simulink library "powerwindowlibsa"  (Simulink 6.0)
settings: Solver=ode45  SolverMode=SingleTasking  StartTime=0.0  StopTime=10.0  RelTol=1e-3
InitFcn:
  | powericon('psbinitsys',bdroot);
libraries: fixpt_lib_4 x2, simulink x2, powerwindowlibsa x1
settings Model: Creator=The MathWorks Inc.  LastModifiedBy=batserve  ExtModeAutoUpdateStatusClock=off
settings OptimizationCC: BooleanDataType=off
settings DebuggingCC: CheckExecutionContextPreStartOutputMsg=on  CheckExecutionContextRuntimeOutputMsg=on  SolverPrmCheckMsg=none
settings HardwareCC: TargetUnknown=on

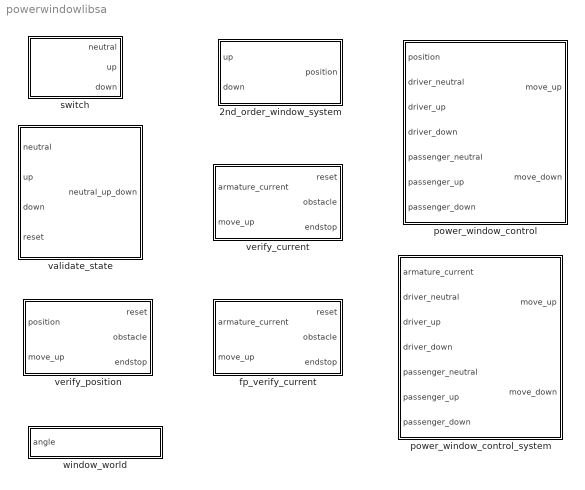
== system powerwindowlibsa ==
  2nd_order_window_system : Subsystem  PropExecContextAcrossSSBoundary=on
  fp_verify_current : Subsystem  AncestorBlock=powerwindowlibsa/verify_current  PropExecContextAcrossSSBoundary=on
  power_window_control : Subsystem  PropExecContextAcrossSSBoundary=on
  power_window_control_system : Subsystem  PropExecContextAcrossSSBoundary=on
  switch : Subsystem  PropExecContextAcrossSSBoundary=on
  validate_state : Subsystem  PropExecContextAcrossSSBoundary=on
  verify_current : Subsystem  AncestorBlock=powerwindowlibsa/power_window_control_system/detect_obstacle_endstop  PropExecContextAcrossSSBoundary=on
  verify_position : Subsystem  AncestorBlock=powerwindowlibsa/detect_obstacle_endstop  PropExecContextAcrossSSBoundary=on
  window_world : Subsystem  AncestorBlock=powerwindowlibsa/window_world  PropExecContextAcrossSSBoundary=on
      settings: OpenFcn=open_system([gcs '/window_world/VR Sink']);
      mask Display: disp(sprintf('Double-click to view scene'))

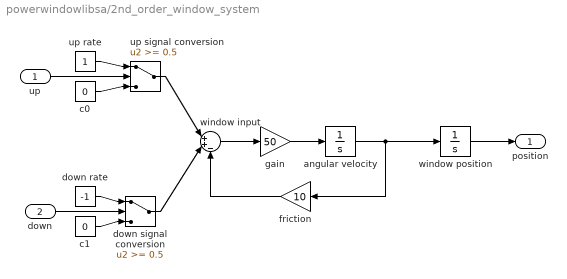
== system powerwindowlibsa/2nd_order_window_system ==
  up : Inport  Port=1  LatchInput=off
  down : Inport  Port=2  LatchInput=off
  angular velocity : Integrator
  c0 : Constant  Value=0
  c1 : Constant  Value=0
  down rate : Constant  Value=-1
  down signal conversion : Switch  Threshold=0.5  SaturateOnIntegerOverflow=on  InputSameDT=on
  friction : Gain  Orientation=left  Gain=10  SaturateOnIntegerOverflow=on
  gain : Gain  Gain=50  SaturateOnIntegerOverflow=on
  up rate : Constant
  up signal conversion : Switch  Threshold=0.5  SaturateOnIntegerOverflow=on  InputSameDT=on
  window input : Sum  Inputs=|++-  SaturateOnIntegerOverflow=on  InputSameDT=on
  window position : Integrator
  position : Outport
  wires:
  down/1 -> down signal conversion/2
  window position/1 -> position/1
  up/1 -> up signal conversion/2
  up rate/1 -> up signal conversion/1
  c0/1 -> up signal conversion/3
  down rate/1 -> down signal conversion/1
  c1/1 -> down signal conversion/3
  up signal conversion/1 -> window input/1
  down signal conversion/1 -> window input/2
  window input/1 -> gain/1
  gain/1 -> angular velocity/1
  angular velocity/1 -> friction/1, window position/1
  friction/1 -> window input/3

== system powerwindowlibsa/fp_verify_current ==
  armature_current : Inport  Port=1  LatchInput=off
  move_up : Inport  Port=2  LatchInput=off
  detect_endstop : Subsystem  PropExecContextAcrossSSBoundary=on
  detect_obstacle : Subsystem  PropExecContextAcrossSSBoundary=on
  either : Logic  Operator=OR
  process_current : Subsystem  PropExecContextAcrossSSBoundary=on
  reset : Outport
  obstacle : Outport  Port=2
  endstop : Outport  Port=3
  wires:
  armature_current/1 -> process_current/1(raw_current)
  detect_obstacle/1(obstacle) -> either/1, obstacle/1
  detect_endstop/1(endstop) -> endstop/1, either/2
  either/1 -> reset/1
  move_up/1 -> detect_obstacle/1(move_up)
  process_current/1(processed_current) -> detect_obstacle/2(armature_current), detect_endstop/1(armature_current)

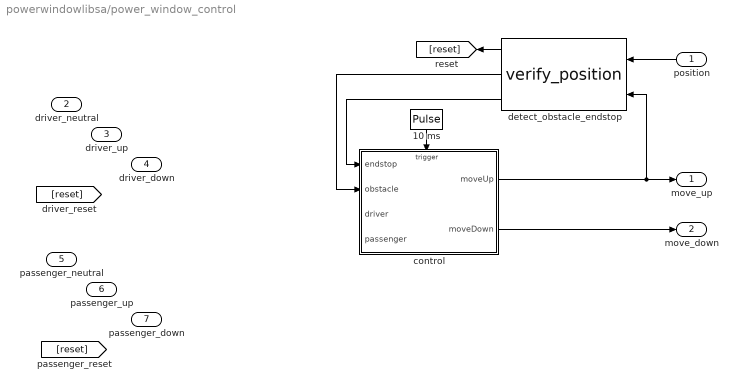
== system powerwindowlibsa/power_window_control ==
  position : Inport  Orientation=left  Port=1  LatchInput=off
  driver_neutral : Inport  Port=2  LatchInput=off
  driver_up : Inport  Port=3  LatchInput=off
  driver_down : Inport  Port=4  LatchInput=off
  passenger_neutral : Inport  Port=5  LatchInput=off
  passenger_up : Inport  Port=6  LatchInput=off
  passenger_down : Inport  Port=7  LatchInput=off
  10 ms : DiscretePulseGenerator  Orientation=down  SampleTime=10e-3
  control : Stateflow chart  TreatAsAtomicUnit=on  PropExecContextAcrossSSBoundary=on
  detect_obstacle_endstop : powerwindowlibsa/verify_position  Orientation=left  AncestorBlock=powerwindowlibsa/detect_obstacle_endstop  SimViewingDevice=off  DataTypeOverride=UseLocalSettings  MinMaxOverflowLogging=UseLocalSettings
      settings: Permissions=ReadWrite  RTWFcnNameOpts=Auto  RTWFileNameOpts=Auto
  move_up : Outport
  move_down : Outport  Port=2
  wires:
  control/2(moveDown) -> move_down/1
  control/1(moveUp) -> move_up/1, detect_obstacle_endstop/2
  10 ms/1 -> control/Trigger
  position/1 -> detect_obstacle_endstop/1
  detect_obstacle_endstop/1 -> [reset]
  detect_obstacle_endstop/3 -> control/1(endstop)
  detect_obstacle_endstop/2 -> control/2(obstacle)

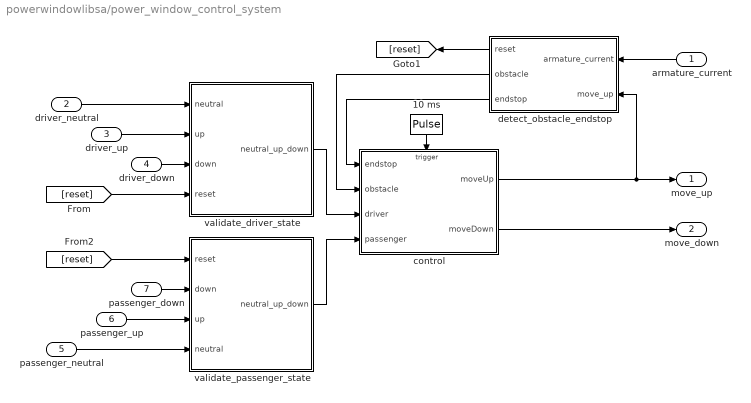
== system powerwindowlibsa/power_window_control_system ==
  armature_current : Inport  Orientation=left  Port=1  LatchInput=off
  driver_neutral : Inport  Port=2  LatchInput=off
  driver_up : Inport  Port=3  LatchInput=off
  driver_down : Inport  Port=4  LatchInput=off
  passenger_neutral : Inport  Port=5  LatchInput=off
  passenger_up : Inport  Port=6  LatchInput=off
  passenger_down : Inport  Port=7  LatchInput=off
  10 ms : DiscretePulseGenerator  Orientation=down  PulseType=Time based  Period=1e-2  SampleTime=1e-3
  control : Stateflow chart  TreatAsAtomicUnit=on  PropExecContextAcrossSSBoundary=on
  detect_obstacle_endstop : Subsystem  Orientation=left  PropExecContextAcrossSSBoundary=on
  validate_driver_state : Subsystem  PropExecContextAcrossSSBoundary=on
  validate_passenger_state : Subsystem  PropExecContextAcrossSSBoundary=on
  move_up : Outport
  move_down : Outport  Port=2
  wires:
  armature_current/1 -> detect_obstacle_endstop/1(armature_current)
  control/2(moveDown) -> move_down/1
  control/1(moveUp) -> detect_obstacle_endstop/2(move_up), move_up/1
  detect_obstacle_endstop/3(endstop) -> control/1(endstop)
  detect_obstacle_endstop/2(obstacle) -> control/2(obstacle)
  validate_passenger_state/1(neutral_up_down) -> control/4(passenger)
  validate_driver_state/1(neutral_up_down) -> control/3(driver)
  10 ms/1 -> control/Trigger
  detect_obstacle_endstop/1(reset) -> [reset]
  [reset] -> validate_passenger_state/1(reset)
  passenger_down/1 -> validate_passenger_state/2(down)
  passenger_up/1 -> validate_passenger_state/3(up)
  passenger_neutral/1 -> validate_passenger_state/4(neutral)
  driver_down/1 -> validate_driver_state/3(down)
  driver_up/1 -> validate_driver_state/2(up)
  driver_neutral/1 -> validate_driver_state/1(neutral)
  [reset] -> validate_driver_state/4(reset)

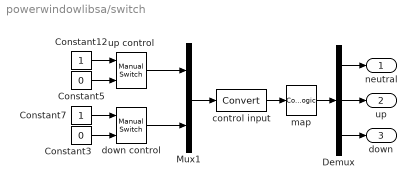
== system powerwindowlibsa/switch ==
  Constant12 : Constant
  Constant3 : Constant  Value=0
  Constant5 : Constant  Value=0
  Constant7 : Constant
  Demux : Demux  Outputs=3
  Mux1 : Mux  Inputs=2
  control input : DataTypeConversion  OutDataTypeMode=boolean  SaturateOnIntegerOverflow=on  RndMeth=Zero
  down control : simulink/Signal Routing/Manual Switch  sw=0  action=0
  map : CombinatorialLogic  TruthTable=[1 0 0;0 0 1;0 1 0;1 0 0]
  up control : simulink/Signal Routing/Manual Switch  sw=0  action=0
  neutral : Outport
  up : Outport  Port=2
  down : Outport  Port=3
  wires:
  Demux/3 -> down/1
  Demux/2 -> up/1
  Demux/1 -> neutral/1
  map/1 -> Demux/1
  up control/1 -> Mux1/1
  Mux1/1 -> control input/1
  down control/1 -> Mux1/2
  Constant3/1 -> down control/2
  Constant7/1 -> down control/1
  Constant5/1 -> up control/2
  Constant12/1 -> up control/1
  control input/1 -> map/1

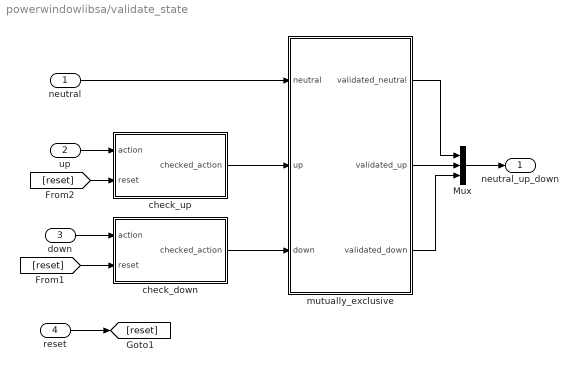
== system powerwindowlibsa/validate_state ==
  neutral : Inport  Port=1  LatchInput=off
  up : Inport  Port=2  LatchInput=off
  down : Inport  Port=3  LatchInput=off
  reset : Inport  Port=4  LatchInput=off
  Mux : Mux  Inputs=3
  check_down : Subsystem  PropExecContextAcrossSSBoundary=on
  check_up : Subsystem  PropExecContextAcrossSSBoundary=on
  mutually_exclusive : Subsystem  PropExecContextAcrossSSBoundary=on
  neutral_up_down : Outport
  wires:
  check_down/1(checked_action) -> mutually_exclusive/3(down)
  mutually_exclusive/3(validated_down) -> Mux/3
  mutually_exclusive/2(validated_up) -> Mux/2
  mutually_exclusive/1(validated_neutral) -> Mux/1
  down/1 -> check_down/1(action)
  up/1 -> check_up/1(action)
  neutral/1 -> mutually_exclusive/1(neutral)
  check_up/1(checked_action) -> mutually_exclusive/2(up)
  [reset] -> check_up/2(reset)
  [reset] -> check_down/2(reset)
  reset/1 -> [reset]
  Mux/1 -> neutral_up_down/1

== system powerwindowlibsa/verify_current ==
  armature_current : Inport  Port=1  LatchInput=off
  move_up : Inport  Port=2  LatchInput=off
  detect_endstop : Subsystem  PropExecContextAcrossSSBoundary=on
  detect_obstacle : Subsystem  PropExecContextAcrossSSBoundary=on
  either : Logic  Operator=OR
  process_current : Subsystem  PropExecContextAcrossSSBoundary=on
  reset : Outport
  obstacle : Outport  Port=2
  endstop : Outport  Port=3
  wires:
  process_current/1(processed_current) -> detect_endstop/1(armature_current), detect_obstacle/2(armature_current)
  move_up/1 -> detect_obstacle/1(move_up)
  either/1 -> reset/1
  detect_endstop/1(endstop) -> either/2, endstop/1
  detect_obstacle/1(obstacle) -> obstacle/1, either/1
  armature_current/1 -> process_current/1(raw_current)

== system powerwindowlibsa/verify_position ==
  position : Inport  Port=1  LatchInput=off
  move_up : Inport  Port=2  LatchInput=off
  detect_endstop : Subsystem  PropExecContextAcrossSSBoundary=on
  detect_obstacle : Subsystem  PropExecContextAcrossSSBoundary=on
  either : Logic  Operator=OR
  reset : Outport
  obstacle : Outport  Port=2
  endstop : Outport  Port=3
  wires:
  move_up/1 -> detect_obstacle/1(move_up)
  position/1 -> detect_endstop/1(position), detect_obstacle/2(position)
  either/1 -> reset/1
  detect_endstop/1(endstop) -> either/2, endstop/1
  detect_obstacle/1(obstacle) -> obstacle/1, either/1

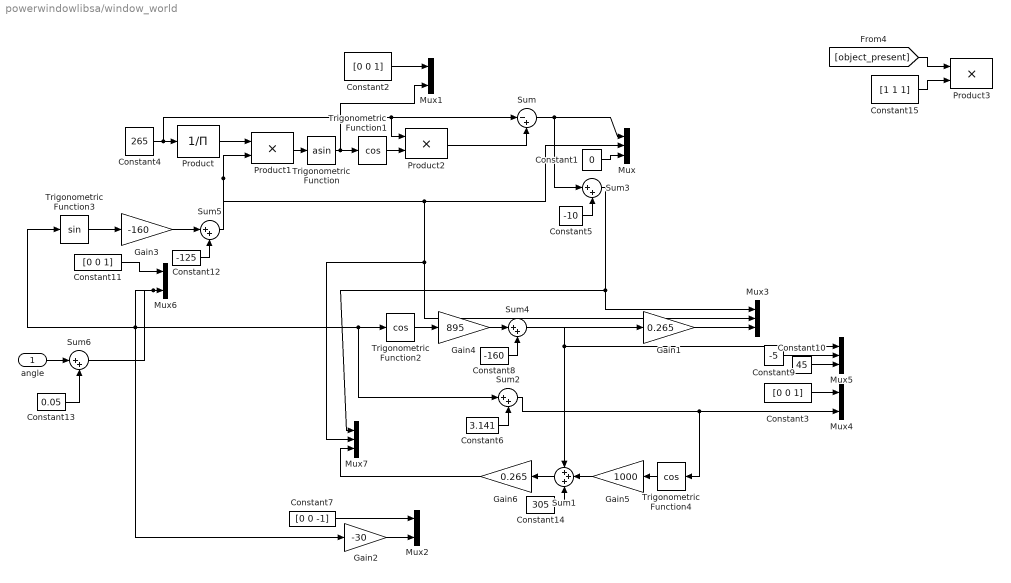
== system powerwindowlibsa/window_world ==
  angle : Inport  Port=1  LatchInput=off
  Constant1 : Constant  Value=0
  Constant10 : Constant  Value=45
  Constant11 : Constant  Value=[0 0 1]
  Constant12 : Constant  Value=-125
  Constant13 : Constant  Value=0.05
  Constant14 : Constant  Value=305
  Constant15 : Constant  Value=[1 1 1]
  Constant2 : Constant  Value=[0 0 1]
  Constant3 : Constant  Value=[0 0 1]
  Constant4 : Constant  Value=265
  Constant5 : Constant  Value=-10
  Constant6 : Constant  Value=3.141
  Constant7 : Constant  Value=[0 0 -1]
  Constant8 : Constant  Value=-160
  Constant9 : Constant  Value=-5
  Gain1 : Gain  Gain=0.265  SaturateOnIntegerOverflow=on
  Gain2 : Gain  Gain=-30  SaturateOnIntegerOverflow=on
  Gain3 : Gain  Gain=-160  SaturateOnIntegerOverflow=on
  Gain4 : Gain  Gain=895  SaturateOnIntegerOverflow=on
  Gain5 : Gain  Orientation=left  Gain=1000  SaturateOnIntegerOverflow=on
  Gain6 : Gain  Orientation=left  Gain=0.265  SaturateOnIntegerOverflow=on
  Mux{,3,5,7} (4 alike) : Mux  Inputs=3
  Mux{1..2,4,6} (4 alike) : Mux  Inputs=2
  Product : Product  Inputs=/  SaturateOnIntegerOverflow=on  InputSameDT=on
  Product1 : Product  SaturateOnIntegerOverflow=on  InputSameDT=on
  Product2 : Product  SaturateOnIntegerOverflow=on  InputSameDT=on
  Product3 : Product  SaturateOnIntegerOverflow=on  InputSameDT=on
  Sum : Sum  Inputs=|-+  SaturateOnIntegerOverflow=on  InputSameDT=on
  Sum1 : Sum  Orientation=left  Inputs=+++  SaturateOnIntegerOverflow=on  InputSameDT=on
  Sum{2..6} (5 alike) : Sum  Inputs=|++  SaturateOnIntegerOverflow=on  InputSameDT=on
  Trigonometric Function : Trigonometry  Operator=asin
  Trigonometric Function1 : Trigonometry  Operator=cos
  Trigonometric Function2 : Trigonometry  Operator=cos
  Trigonometric Function3 : Trigonometry
  Trigonometric Function4 : Trigonometry  Orientation=left  Operator=cos
  wires:
  Constant5/1 -> Sum3/2
  Sum3/1 -> Mux7/1, Mux3/1
  Constant14/1 -> Sum1/3
  Gain6/1 -> Mux7/3
  Sum1/1 -> Gain6/1
  Gain5/1 -> Sum1/2
  Trigonometric Function4/1 -> Gain5/1
  Gain1/1 -> Mux3/3
  Constant7/1 -> Mux2/1
  Gain2/1 -> Mux2/2
  Sum5/1 -> Mux7/2, Mux3/2, Mux/2, Product1/2
  Gain3/1 -> Sum5/1
  Constant12/1 -> Sum5/2
  Constant11/1 -> Mux6/1
  Trigonometric Function3/1 -> Gain3/1
  Constant8/1 -> Sum4/2
  Sum4/1 -> Sum1/1, Mux5/1, Gain1/1
  Gain4/1 -> Sum4/1
  Trigonometric Function2/1 -> Gain4/1
  Constant10/1 -> Mux5/3
  Constant9/1 -> Mux5/2
  Constant6/1 -> Sum2/2
  Sum2/1 -> Trigonometric Function4/1, Mux4/2
  Constant3/1 -> Mux4/1
  Sum/1 -> Sum3/1, Mux/1
  Product2/1 -> Sum/2
  Trigonometric Function1/1 -> Product2/2
  Trigonometric Function/1 -> Mux1/2, Trigonometric Function1/1
  Product1/1 -> Trigonometric Function/1
  Product/1 -> Product1/1
  Constant4/1 -> Sum/1, Product2/1, Product/1
  Constant2/1 -> Mux1/1
  Constant1/1 -> Mux/3
  Sum6/1 -> Mux6/2, Gain2/1, Trigonometric Function2/1, Sum2/1, Trigonometric Function3/1
  angle/1 -> Sum6/1
  Constant13/1 -> Sum6/2
  Constant15/1 -> Product3/2
  [object_present] -> Product3/1

== system powerwindowlibsa/fp_verify_current/detect_endstop ==
  armature_current : Inport  Port=1  LatchInput=off
  current_limit : fixpt_lib_4/Logic & Comparison/Compare To Constant  relop=>  const=15
  passenger control : DataTypeConversion  OutDataTypeMode=boolean  SaturateOnIntegerOverflow=on  RndMeth=Zero
  endstop : Outport
  wires:
  passenger control/1 -> endstop/1
  current_limit/1 -> passenger control/1
  armature_current/1 -> current_limit/1

== system powerwindowlibsa/fp_verify_current/detect_obstacle ==
  move_up : Inport  Orientation=left  Port=1  LatchInput=off
  armature_current : Inport  Port=2  LatchInput=off
  10 ms : DiscretePulseGenerator  Orientation=down  SampleTime=10e-3
  Multiply : Product  Orientation=up  Inputs=**  OutDataType=sfix(8)  OutScaling=2^-5
  break dependency : UnitDelay  Orientation=left  SampleTime=0.01
  current_limit : fixpt_lib_4/Logic & Comparison/Compare To Constant  relop=>  const=1.1
  delay_detection : Stateflow chart  Orientation=left  TreatAsAtomicUnit=on  PropExecContextAcrossSSBoundary=on
  passenger control : DataTypeConversion  Orientation=up  OutDataTypeMode=boolean  SaturateOnIntegerOverflow=on  RndMeth=Zero
  obstacle : Outport  Orientation=up
  wires:
  passenger control/1 -> obstacle/1
  break dependency/1 -> delay_detection/1(move_up)
  10 ms/1 -> delay_detection/Trigger
  Multiply/1 -> passenger control/1
  move_up/1 -> break dependency/1
  armature_current/1 -> current_limit/1
  delay_detection/1(detect) -> Multiply/2
  current_limit/1 -> Multiply/1

== system powerwindowlibsa/fp_verify_current/process_current ==
  raw_current : Inport  Port=1  LatchInput=off
  3.5 / (2^(bits-1)) : Gain  Gain=0.02734375  ParameterDataType=sfix( 8 )  ParameterScaling=2^-12  OutDataTypeMode=Specify via dialog  OutScaling=2^-6
  Abs : Abs
  gain : Gain  Gain=5  ParameterDataType=sfix( 8 )  ParameterScaling=2^-4  OutDataTypeMode=Specify via dialog  OutScaling=2^-5
  processed_current : Outport
  wires:
  raw_current/1 -> 3.5 / (2^(bits-1))/1
  Abs/1 -> processed_current/1
  gain/1 -> Abs/1
  3.5 / (2^(bits-1))/1 -> gain/1

== system powerwindowlibsa/power_window_control_system/detect_obstacle_endstop ==
  armature_current : Inport  Port=1  LatchInput=off
  move_up : Inport  Port=2  LatchInput=off
  Abs : Abs  SaturateOnIntegerOverflow=on
  detect_endstop : Subsystem  PropExecContextAcrossSSBoundary=on
  detect_obstacle : Subsystem  PropExecContextAcrossSSBoundary=on
  either : Logic  Operator=OR
  reset : Outport
  obstacle : Outport  Port=2
  endstop : Outport  Port=3
  wires:
  detect_obstacle/1(obstacle) -> either/1, obstacle/1
  detect_endstop/1(endstop) -> endstop/1, either/2
  either/1 -> reset/1
  armature_current/1 -> Abs/1
  move_up/1 -> detect_obstacle/1(move_up)
  Abs/1 -> detect_obstacle/2(armature_current), detect_endstop/1(armature_current)

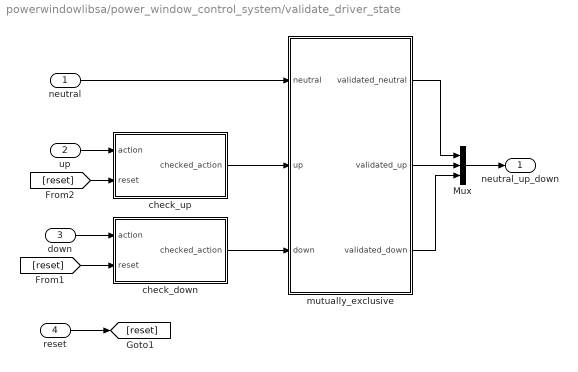
== system powerwindowlibsa/power_window_control_system/validate_driver_state ==
  neutral : Inport  Port=1  LatchInput=off
  up : Inport  Port=2  LatchInput=off
  down : Inport  Port=3  LatchInput=off
  reset : Inport  Port=4  LatchInput=off
  Mux : Mux  Inputs=3
  check_down : Subsystem  PropExecContextAcrossSSBoundary=on
  check_up : Subsystem  PropExecContextAcrossSSBoundary=on
  mutually_exclusive : Subsystem  PropExecContextAcrossSSBoundary=on
  neutral_up_down : Outport
  wires:
  check_down/1(checked_action) -> mutually_exclusive/3(down)
  mutually_exclusive/3(validated_down) -> Mux/3
  mutually_exclusive/2(validated_up) -> Mux/2
  mutually_exclusive/1(validated_neutral) -> Mux/1
  down/1 -> check_down/1(action)
  up/1 -> check_up/1(action)
  neutral/1 -> mutually_exclusive/1(neutral)
  check_up/1(checked_action) -> mutually_exclusive/2(up)
  [reset] -> check_up/2(reset)
  [reset] -> check_down/2(reset)
  reset/1 -> [reset]
  Mux/1 -> neutral_up_down/1

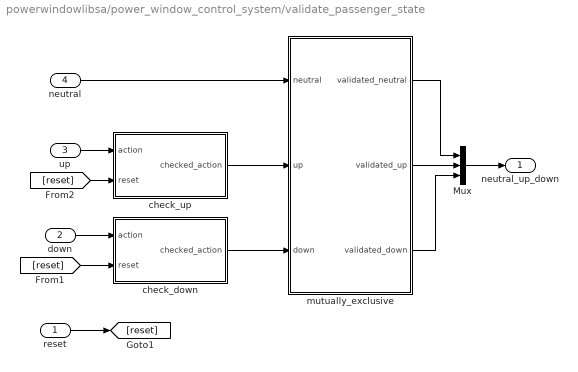
== system powerwindowlibsa/power_window_control_system/validate_passenger_state ==
  reset : Inport  Port=1  LatchInput=off
  down : Inport  Port=2  LatchInput=off
  up : Inport  Port=3  LatchInput=off
  neutral : Inport  Port=4  LatchInput=off
  Mux : Mux  Inputs=3
  check_down : Subsystem  PropExecContextAcrossSSBoundary=on
  check_up : Subsystem  PropExecContextAcrossSSBoundary=on
  mutually_exclusive : Subsystem  PropExecContextAcrossSSBoundary=on
  neutral_up_down : Outport
  wires:
  Mux/1 -> neutral_up_down/1
  reset/1 -> [reset]
  [reset] -> check_down/2(reset)
  [reset] -> check_up/2(reset)
  check_up/1(checked_action) -> mutually_exclusive/2(up)
  neutral/1 -> mutually_exclusive/1(neutral)
  up/1 -> check_up/1(action)
  down/1 -> check_down/1(action)
  mutually_exclusive/1(validated_neutral) -> Mux/1
  mutually_exclusive/2(validated_up) -> Mux/2
  mutually_exclusive/3(validated_down) -> Mux/3
  check_down/1(checked_action) -> mutually_exclusive/3(down)

== system powerwindowlibsa/validate_state/check_down ==
  action : Inport  Port=1  LatchInput=off
  reset : Inport  Port=2  LatchInput=off
  allow_action : Logic
  overrule : Logic  Operator=NOT
  checked_action : Outport
  wires:
  overrule/1 -> allow_action/2
  action/1 -> allow_action/1
  allow_action/1 -> checked_action/1
  reset/1 -> overrule/1

== system powerwindowlibsa/validate_state/check_up ==
  action : Inport  Port=1  LatchInput=off
  reset : Inport  Port=2  LatchInput=off
  allow_action : Logic
  overrule : Logic  Operator=NOT
  checked_action : Outport
  wires:
  reset/1 -> overrule/1
  allow_action/1 -> checked_action/1
  action/1 -> allow_action/1
  overrule/1 -> allow_action/2

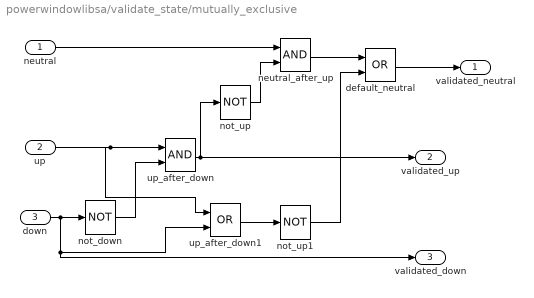
== system powerwindowlibsa/validate_state/mutually_exclusive ==
  neutral : Inport  Port=1  LatchInput=off
  up : Inport  Port=2  LatchInput=off
  down : Inport  Port=3  LatchInput=off
  default_neutral : Logic  Operator=OR
  neutral_after_up : Logic
  not_down : Logic  Operator=NOT
  not_up : Logic  Operator=NOT
  not_up1 : Logic  Operator=NOT
  up_after_down : Logic
  up_after_down1 : Logic  Operator=OR
  validated_neutral : Outport
  validated_up : Outport  Port=2
  validated_down : Outport  Port=3
  wires:
  not_up1/1 -> default_neutral/2
  default_neutral/1 -> validated_neutral/1
  neutral_after_up/1 -> default_neutral/1
  up_after_down1/1 -> not_up1/1
  up/1 -> up_after_down1/1, up_after_down/1
  neutral/1 -> neutral_after_up/1
  down/1 -> validated_down/1, up_after_down1/2, not_down/1
  not_up/1 -> neutral_after_up/2
  up_after_down/1 -> validated_up/1, not_up/1
  not_down/1 -> up_after_down/2

== system powerwindowlibsa/verify_current/detect_endstop ==
  armature_current : Inport  Port=1  LatchInput=off
  Constant6 : Constant  Value=15
  current_limit : RelationalOperator  Operator=>  InputSameDT=on
  passenger control : DataTypeConversion  OutDataTypeMode=boolean  SaturateOnIntegerOverflow=on  RndMeth=Zero
  endstop : Outport
  wires:
  Constant6/1 -> current_limit/2
  armature_current/1 -> current_limit/1
  current_limit/1 -> passenger control/1
  passenger control/1 -> endstop/1

== system powerwindowlibsa/verify_current/detect_obstacle ==
  move_up : Inport  Orientation=left  Port=1  LatchInput=off
  armature_current : Inport  Port=2  LatchInput=off
  10 ms1 : DiscretePulseGenerator  Orientation=down  SampleTime=10e-3
  Constant1 : Constant  Value=1.2
  Product : Product  Orientation=up  SaturateOnIntegerOverflow=on  InputSameDT=on
  break dependency : UnitDelay  Orientation=left  SampleTime=0.01
  delay_detection : Stateflow chart  Orientation=left  TreatAsAtomicUnit=on  PropExecContextAcrossSSBoundary=on
  object : RelationalOperator  Operator=>  InputSameDT=on
  passenger control : DataTypeConversion  Orientation=up  OutDataTypeMode=boolean  SaturateOnIntegerOverflow=on  RndMeth=Zero
  obstacle : Outport  Orientation=up
  wires:
  Constant1/1 -> object/2
  object/1 -> Product/1
  delay_detection/1(detect) -> Product/2
  armature_current/1 -> object/1
  move_up/1 -> break dependency/1
  Product/1 -> passenger control/1
  10 ms1/1 -> delay_detection/Trigger
  break dependency/1 -> delay_detection/1(move_up)
  passenger control/1 -> obstacle/1

== system powerwindowlibsa/verify_current/process_current ==
  raw_current : Inport  Port=1  LatchInput=off
  Abs : Abs  SaturateOnIntegerOverflow=on
  processed_current : Outport
  wires:
  Abs/1 -> processed_current/1
  raw_current/1 -> Abs/1

== system powerwindowlibsa/verify_position/detect_endstop ==
  position : Inport  Port=1  LatchInput=off
  Constant6 : Constant  Value=0.4
  current_limit : RelationalOperator  Operator=>  InputSameDT=on
  passenger control : DataTypeConversion  OutDataTypeMode=boolean  SaturateOnIntegerOverflow=on  RndMeth=Zero
  endstop : Outport
  wires:
  Constant6/1 -> current_limit/2
  position/1 -> current_limit/1
  current_limit/1 -> passenger control/1
  passenger control/1 -> endstop/1

== system powerwindowlibsa/verify_position/detect_obstacle ==
  move_up : Inport  Orientation=left  Port=1  LatchInput=off
  position : Inport  Port=2  LatchInput=off
  Break Dependency : Memory  Orientation=left
  Constant1 : Constant  Value=0.3
  Product : Product  Orientation=up  SaturateOnIntegerOverflow=on  InputSameDT=on
  object : RelationalOperator  Operator=>  InputSameDT=on
  passenger control : DataTypeConversion  Orientation=up  OutDataTypeMode=boolean  SaturateOnIntegerOverflow=on  RndMeth=Zero
  obstacle : Outport  Orientation=up
  wires:
  Constant1/1 -> object/2
  object/1 -> Product/1
  position/1 -> object/1
  move_up/1 -> Break Dependency/1
  Break Dependency/1 -> Product/2
  Product/1 -> passenger control/1
  passenger control/1 -> obstacle/1

== system powerwindowlibsa/power_window_control_system/detect_obstacle_endstop/detect_endstop ==
  armature_current : Inport  Port=1  LatchInput=off
  Constant6 : Constant  Value=15
  current_limit : RelationalOperator  Operator=>  InputSameDT=on
  endstop : Outport
  wires:
  current_limit/1 -> endstop/1
  armature_current/1 -> current_limit/1
  Constant6/1 -> current_limit/2

== system powerwindowlibsa/power_window_control_system/detect_obstacle_endstop/detect_obstacle ==
  move_up : Inport  Orientation=left  Port=1  LatchInput=off
  armature_current : Inport  Port=2  LatchInput=off
  Constant1 : Constant  Value=1.6
  Product : Product  Orientation=up  SaturateOnIntegerOverflow=on  InputSameDT=on
  break dependency : UnitDelay  Orientation=left  SampleTime=0.01
  delay 500 ms : Subsystem  Orientation=left  TreatAsAtomicUnit=on  PropExecContextAcrossSSBoundary=on
  object : RelationalOperator  Operator=>  InputSameDT=on
  obstacle : Outport  Orientation=up
  wires:
  break dependency/1 -> delay 500 ms/Enable
  Product/1 -> obstacle/1
  move_up/1 -> break dependency/1
  armature_current/1 -> object/1
  delay 500 ms/1(step) -> Product/2
  object/1 -> Product/1
  Constant1/1 -> object/2

== system powerwindowlibsa/power_window_control_system/validate_driver_state/check_down ==
  action : Inport  Port=1  LatchInput=off
  reset : Inport  Port=2  LatchInput=off
  allow_action : Logic
  overrule : Logic  Operator=NOT
  checked_action : Outport
  wires:
  overrule/1 -> allow_action/2
  action/1 -> allow_action/1
  allow_action/1 -> checked_action/1
  reset/1 -> overrule/1

== system powerwindowlibsa/power_window_control_system/validate_driver_state/check_up ==
  action : Inport  Port=1  LatchInput=off
  reset : Inport  Port=2  LatchInput=off
  allow_action : Logic
  overrule : Logic  Operator=NOT
  checked_action : Outport
  wires:
  reset/1 -> overrule/1
  allow_action/1 -> checked_action/1
  action/1 -> allow_action/1
  overrule/1 -> allow_action/2

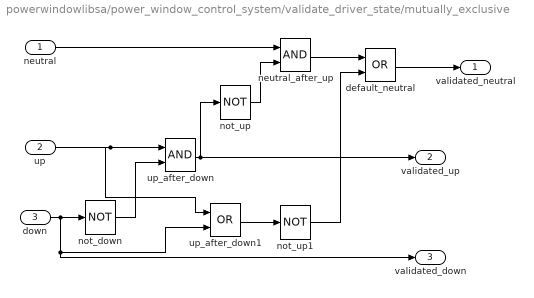
== system powerwindowlibsa/power_window_control_system/validate_driver_state/mutually_exclusive ==
  neutral : Inport  Port=1  LatchInput=off
  up : Inport  Port=2  LatchInput=off
  down : Inport  Port=3  LatchInput=off
  default_neutral : Logic  Operator=OR
  neutral_after_up : Logic
  not_down : Logic  Operator=NOT
  not_up : Logic  Operator=NOT
  not_up1 : Logic  Operator=NOT
  up_after_down : Logic
  up_after_down1 : Logic  Operator=OR
  validated_neutral : Outport
  validated_up : Outport  Port=2
  validated_down : Outport  Port=3
  wires:
  not_up1/1 -> default_neutral/2
  default_neutral/1 -> validated_neutral/1
  neutral_after_up/1 -> default_neutral/1
  up_after_down1/1 -> not_up1/1
  up/1 -> up_after_down1/1, up_after_down/1
  neutral/1 -> neutral_after_up/1
  down/1 -> validated_down/1, up_after_down1/2, not_down/1
  not_up/1 -> neutral_after_up/2
  up_after_down/1 -> validated_up/1, not_up/1
  not_down/1 -> up_after_down/2

== system powerwindowlibsa/power_window_control_system/validate_passenger_state/check_down ==
  action : Inport  Port=1  LatchInput=off
  reset : Inport  Port=2  LatchInput=off
  allow_action : Logic
  overrule : Logic  Operator=NOT
  checked_action : Outport
  wires:
  reset/1 -> overrule/1
  allow_action/1 -> checked_action/1
  action/1 -> allow_action/1
  overrule/1 -> allow_action/2

== system powerwindowlibsa/power_window_control_system/validate_passenger_state/check_up ==
  action : Inport  Port=1  LatchInput=off
  reset : Inport  Port=2  LatchInput=off
  allow_action : Logic
  overrule : Logic  Operator=NOT
  checked_action : Outport
  wires:
  overrule/1 -> allow_action/2
  action/1 -> allow_action/1
  allow_action/1 -> checked_action/1
  reset/1 -> overrule/1

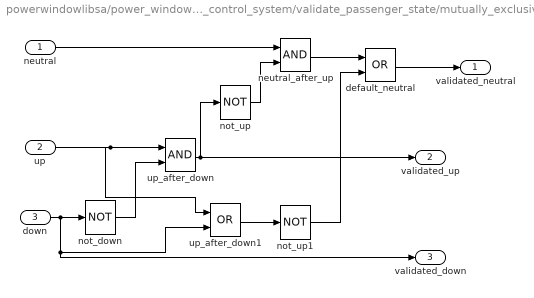
== system powerwindowlibsa/power_window_control_system/validate_passenger_state/mutually_exclusive ==
  neutral : Inport  Port=1  LatchInput=off
  up : Inport  Port=2  LatchInput=off
  down : Inport  Port=3  LatchInput=off
  default_neutral : Logic  Operator=OR
  neutral_after_up : Logic
  not_down : Logic  Operator=NOT
  not_up : Logic  Operator=NOT
  not_up1 : Logic  Operator=NOT
  up_after_down : Logic
  up_after_down1 : Logic  Operator=OR
  validated_neutral : Outport
  validated_up : Outport  Port=2
  validated_down : Outport  Port=3
  wires:
  not_down/1 -> up_after_down/2
  up_after_down/1 -> not_up/1, validated_up/1
  not_up/1 -> neutral_after_up/2
  down/1 -> not_down/1, up_after_down1/2, validated_down/1
  neutral/1 -> neutral_after_up/1
  up/1 -> up_after_down/1, up_after_down1/1
  up_after_down1/1 -> not_up1/1
  neutral_after_up/1 -> default_neutral/1
  default_neutral/1 -> validated_neutral/1
  not_up1/1 -> default_neutral/2

== system powerwindowlibsa/power_window_control_system/detect_obstacle_endstop/detect_obstacle/delay 500 ms ==
  Enable : EnablePort  StatesWhenEnabling=reset
  Constant : Constant
  Constant1 : Constant  Value=0.5
  Integrator : Integrator
  Relational Operator : RelationalOperator  Operator=>  InputSameDT=on
  step : Outport  OutputWhenDisabled=reset  InitialOutput=0
  wires:
  Relational Operator/1 -> step/1
  Constant1/1 -> Relational Operator/2
  Integrator/1 -> Relational Operator/1
  Constant/1 -> Integrator/1

== stateflow chart power_window_control_system/control ==
  settings: executeAtInitialization=1
  state emergencyDown
    entry:
    moveUp = 0;
    moveDown = 1;
  state safe
    state driverUp
      entry: moveUp = 1;
      exit: moveUp = 0;
      state iniDriverUp
      state DriverUp
      state autoDriverUp
      iniDriverUp -> (junction 26) : after(100,ticks)
      (junction 26) -> DriverUp
      (junction 26) -> autoDriverUp : [driver[1]]
    state driverDown
      entry: moveDown = 1;
      exit: moveDown = 0;
      state iniDriverDown
      state DriverDown
      state autoDriverDown
      iniDriverDown -> (junction 25) : after(100,ticks)
      (junction 25) -> autoDriverDown : [driver[1]]
      (junction 25) -> DriverDown
    state driverNeutral
      entry:
      moveUp = 0;
      moveDown = 0;
      state passengerneutral
        entry:
        moveUp = 0;
        moveDown = 0;
      state passengerUp
        entry: moveUp = 1;
        exit: moveUp = 0;
        state iniPassengerUp
        state PassengerUp
        state autoPassengerUp
        (junction 24) -> PassengerUp
        (junction 24) -> autoPassengerUp : [passenger[1]]
        iniPassengerUp -> (junction 24) : after(100,ticks)
      state passengerDown
        entry: moveDown = 1;
        exit: moveDown = 0;
        state iniPassengerDown
        state passengerDown
        state autoPassengerDown
        (junction 23) -> autoPassengerDown : [passenger[1]]
        iniPassengerDown -> (junction 23) : after(100,ticks)
        (junction 23) -> safe.driverNeutral.passengerDown.passengerDown
      safe.driverNeutral.passengerDown.passengerDown -> passengerneutral : [passenger[1]]
      safe.driverNeutral.passengerDown -> passengerneutral : [endstop]
      PassengerUp -> passengerneutral : [passenger[1]]
      passengerUp -> passengerneutral : [endstop]
      passengerneutral -> iniPassengerDown : [passenger[3]]
      passengerneutral -> iniPassengerUp : [passenger[2]]
      safe.driverNeutral.passengerDown -> PassengerUp : [passenger[2]]
      passengerUp -> safe.driverNeutral.passengerDown.passengerDown : [passenger[3]]
      (default) -> passengerneutral
    driverNeutral -> iniDriverDown : [driver[3]]
    driverUp -> DriverDown : [driver[3]]
    driverDown -> DriverUp : [driver[2]]
    driverNeutral -> iniDriverUp : [driver[2]]
    DriverDown -> driverNeutral : [driver[1]]
    DriverUp -> driverNeutral : [driver[1]]
    driverDown -> driverNeutral : [endstop]
    driverUp -> driverNeutral : [endstop]
    (default) -> driverNeutral
  emergencyDown -> passengerneutral : [endstop | after(100,ticks)]
  safe -> emergencyDown : [obstacle]
  (default) -> safe
  data: moveUp output double; moveDown output double; endstop input boolean; obstacle input boolean; driver input boolean size=3; passenger input boolean size=3
  events: ticks input RISING_EDGE_EVENT

== stateflow chart power_window_control/control ==
  settings: executeAtInitialization=1
  state emergencyDown
    entry:
    moveUp = 0;
    moveDown = 1;
  state safe
    state driverUp
      entry: moveUp = 1;
      exit: moveUp = 0;
      state iniDriverUp
      state DriverUp
      state autoDriverUp
      iniDriverUp -> (junction 92) : after(100,ticks)
      (junction 92) -> DriverUp
      (junction 92) -> autoDriverUp : [driver[1]]
    state driverDown
      entry: moveDown = 1;
      exit: moveDown = 0;
      state iniDriverDown
      state DriverDown
      state autoDriverDown
      iniDriverDown -> (junction 91) : after(100,ticks)
      (junction 91) -> autoDriverDown : [driver[1]]
      (junction 91) -> DriverDown
    state driverNeutral
      entry:
      moveUp = 0;
      moveDown = 0;
      state passengerneutral
        entry:
        moveUp = 0;
        moveDown = 0;
      state passengerUp
        entry: moveUp = 1;
        exit: moveUp = 0;
        state iniPassengerUp
        state PassengerUp
        state autoPassengerUp
        (junction 90) -> PassengerUp
        (junction 90) -> autoPassengerUp : [passenger[1]]
        iniPassengerUp -> (junction 90) : after(100,ticks)
      state passengerDown
        entry: moveDown = 1;
        exit: moveDown = 0;
        state iniPassengerDown
        state passengerDown
        state autoPassengerDown
        (junction 89) -> autoPassengerDown : [passenger[1]]
        iniPassengerDown -> (junction 89) : after(100,ticks)
        (junction 89) -> safe.driverNeutral.passengerDown.passengerDown
      safe.driverNeutral.passengerDown.passengerDown -> passengerneutral : [passenger[1]]
      safe.driverNeutral.passengerDown -> passengerneutral : [endstop]
      PassengerUp -> passengerneutral : [passenger[1]]
      passengerUp -> passengerneutral : [endstop]
      passengerneutral -> iniPassengerDown : [passenger[3]]
      passengerneutral -> iniPassengerUp : [passenger[2]]
      safe.driverNeutral.passengerDown -> PassengerUp : [passenger[2]]
      passengerUp -> safe.driverNeutral.passengerDown.passengerDown : [passenger[3]]
      (default) -> passengerneutral
    driverNeutral -> iniDriverDown : [driver[3]]
    driverUp -> DriverDown : [driver[3]]
    driverDown -> DriverUp : [driver[2]]
    driverNeutral -> iniDriverUp : [driver[2]]
    DriverDown -> driverNeutral : [driver[1]]
    DriverUp -> driverNeutral : [driver[1]]
    driverDown -> driverNeutral : [endstop]
    driverUp -> driverNeutral : [endstop]
    (default) -> driverNeutral
  emergencyDown -> passengerneutral : [endstop | after(100,ticks)]
  safe -> emergencyDown : [obstacle]
  (default) -> safe
  data: moveUp output double; moveDown output double; endstop input boolean; obstacle input boolean; driver input boolean size=3; passenger input boolean size=3
  events: ticks input EITHER_EDGE_EVENT

== stateflow chart verify_current/detect_obstacle/delay_detection ==
  settings: executeAtInitialization=1
  state detect
  state off
  state hold
  (default) -> off
  off -> hold : [move_up]
  detect -> off : [~move_up]
  hold -> detect : [after(100,ticks)]
  hold -> off : [~move_up]
  data: detect output State; move_up input boolean
  events: ticks input EITHER_EDGE_EVENT

== stateflow chart fp_verify_current/detect_obstacle/delay_detection ==
  settings: executeAtInitialization=1
  state detect
  state off
  state hold
  (default) -> off
  off -> hold : [move_up]
  detect -> off : [~move_up]
  hold -> detect : [after(100,ticks)]
  hold -> off : [~move_up]
  data: detect output State; move_up input boolean
  events: ticks input EITHER_EDGE_EVENT
